simulink model "p4"  (R2022a)
settings: Solver=VariableStepAuto  StartTime=0.0  StopTime=1700  RelTol=1e-3
values from neighbouring files (symbols this model uses):
  fs = 1/3    (= 0.333333333333)    [p2.m]
settings Model: Creator=jorch  LastModifiedBy=jorch

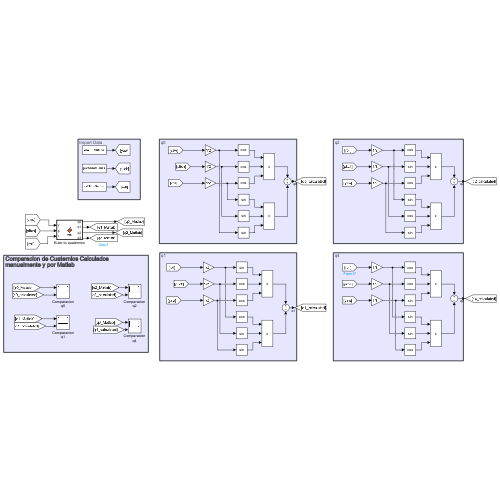
[thumbnail: Simulink's stored preview of the top-level diagram]
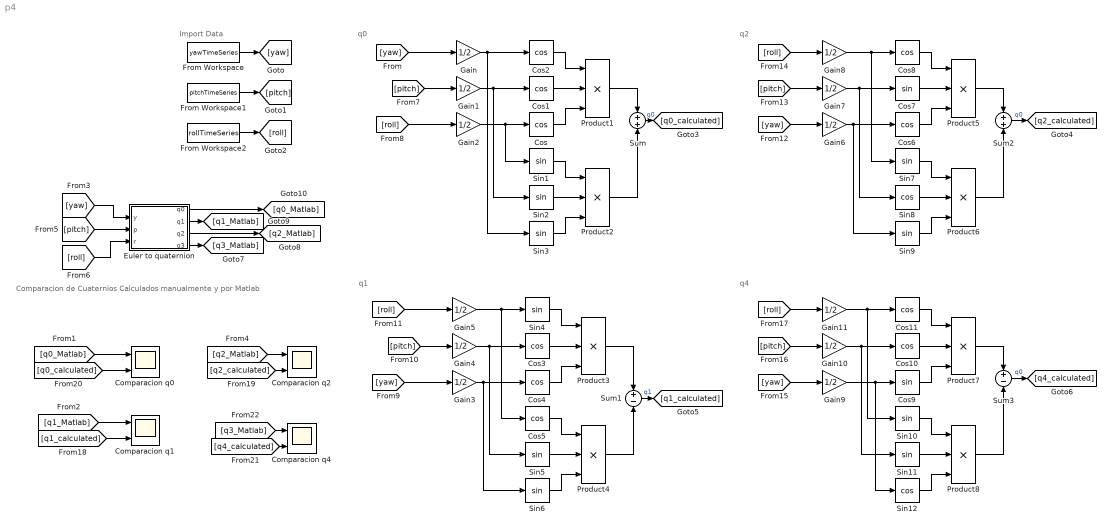
== system p4 ==
  note: Comparacion de Cuaternios Calculados
      | manualmente y por Matlab
  note: Import Data
  note: q4
  note: q2
  note: q0
  note: q1
  Comparacion q{0..2,4} (4 alike) : Scope  NumInputPorts=2
  Cos{,1..6,8,10..11} (10 alike) : Trigonometry  Operator=cos
  Cos7 : Trigonometry
  Cos9 : Trigonometry
  Euler to quaternion : MATLAB Function  TreatAsAtomicUnit=on
  From Workspace : FromWorkspace  VariableName=yawTimeSeries  SampleTime=fs
  From Workspace1 : FromWorkspace  VariableName=pitchTimeSeries  SampleTime=fs
  From Workspace2 : FromWorkspace  VariableName=rollTimeSeries  SampleTime=fs
  Gain{,1..11} (12 alike) : Gain  Gain=1/2
  Product{1..8} (8 alike) : Product  Inputs=3
  Sin{1..7,9..11} (10 alike) : Trigonometry
  Sin12 : Trigonometry  Operator=cos
  Sin8 : Trigonometry  Operator=cos
  Sum : Sum  Inputs=+|+
  Sum1 : Sum  Inputs=+|-
  Sum2 : Sum  Inputs=+|+
  Sum3 : Sum  Inputs=+|-
  wires:
  From Workspace/1 -> [yaw]
  [yaw] -> Euler to quaternion/1(y)
  [pitch] -> Euler to quaternion/2(p)
  [roll] -> Euler to quaternion/3(r)
  From Workspace1/1 -> [pitch]
  From Workspace2/1 -> [roll]
  Gain4/1 -> Sin5/1, Cos3/1
  Gain3/1 -> Cos4/1, Sin6/1
  [yaw] -> Gain3/1
  Product3/1 -> Sum1/1
  Sin6/1 -> Product4/3
  Product4/1 -> Sum1/2
  Gain5/1 -> Cos5/1, Sin4/1
  Cos5/1 -> Product4/1
  Cos3/1 -> Product3/2
  Sin5/1 -> Product4/2
  Sin4/1 -> Product3/1
  Cos4/1 -> Product3/3
  [pitch] -> Gain4/1
  [roll] -> Gain5/1
  Gain2/1 -> Sin1/1, Cos/1
  [yaw] -> Gain/1
  [roll] -> Gain2/1
  Gain1/1 -> Cos1/1, Sin2/1
  Cos2/1 -> Product1/1
  Sin3/1 -> Product2/3
  Product2/1 -> Sum/2
  Gain/1 -> Sin3/1, Cos2/1
  Product1/1 -> Sum/1
  Sin2/1 -> Product2/2
  Cos1/1 -> Product1/2
  Sin1/1 -> Product2/1
  Cos/1 -> Product1/3
  [pitch] -> Gain1/1
  Gain8/1 -> Sin7/1, Cos8/1
  Sin7/1 -> Product6/1
  Cos8/1 -> Product5/1
  Cos6/1 -> Product5/3
  [pitch] -> Gain7/1
  Gain6/1 -> Cos6/1, Sin9/1
  [yaw] -> Gain6/1
  Sin8/1 -> Product6/2
  Cos7/1 -> Product5/2
  Sin9/1 -> Product6/3
  Product5/1 -> Sum2/1
  [roll] -> Gain8/1
  Product6/1 -> Sum2/2
  Gain7/1 -> Cos7/1, Sin8/1
  Sin10/1 -> Product8/1
  Cos11/1 -> Product7/1
  Cos9/1 -> Product7/3
  [pitch] -> Gain10/1
  Sin12/1 -> Product8/3
  Gain11/1 -> Sin10/1, Cos11/1
  Sin11/1 -> Product8/2
  Cos10/1 -> Product7/2
  [roll] -> Gain11/1
  Product7/1 -> Sum3/1
  Product8/1 -> Sum3/2
  Gain10/1 -> Sin11/1, Cos10/1
  Gain9/1 -> Sin12/1, Cos9/1
  [yaw] -> Gain9/1
  Sum/1 -> [q0_calculated]  "q0"
  Sum2/1 -> [q2_calculated]  "q0"
  Sum1/1 -> [q1_calculated]  "q1"
  Sum3/1 -> [q4_calculated]  "q0"
  Euler to quaternion/4(q3) -> [q3_Matlab]
  Euler to quaternion/2(q1) -> [q1_Matlab]
  Euler to quaternion/1(q0) -> [q0_Matlab]
  Euler to quaternion/3(q2) -> [q2_Matlab]
  [q0_Matlab] -> Comparacion q0/1
  [q0_calculated] -> Comparacion q0/2
  [q2_calculated] -> Comparacion q2/2
  [q2_Matlab] -> Comparacion q2/1
  [q1_calculated] -> Comparacion q1/2
  [q1_Matlab] -> Comparacion q1/1
  [q4_calculated] -> Comparacion q4/2
  [q3_Matlab] -> Comparacion q4/1

== matlab function p4/Euler to quaternion ==
  data: y input; q0 output; p input; r input; q1 output; q2 output; q3 output
function [q0, q1, q2, q3] = fcn(y,p,r)
u = [y, p, r];

q = eul2quat(u);

q0 = q(1);
q1 = q(2);
q2 = q(3);
q3 = q(4);
end
